simulink model "laneChangeOutputFeedback"  (R2019a)
settings: Solver=VariableStepAuto  StartTime=0.0  StopTime=60  RelTol=1e-3
values from neighbouring files (symbols this model uses):
  A = [-2 -timeHeadway 0]    [Controller.m]    (also in SimulinkScenario.m = [1 0 0;beta1 1 0; beta0 beta1 1; 0 beta0 beta1; 0 0 beta0])
  B = [0; b1; 0; b2]    [SimulinkScenario.m]
  C = [1 timeHeadway 0; 0 1 timeHeadway; 0 0 1]    [Controller.m]    (also in SimulinkScenario.m = [1 0 0 0])
  Cf = 12e3    (= 12000)    [sim_parameters.m]
  Cr = 11e3    (= 11000)    [sim_parameters.m]
  inputTau = 1    [SimulinkScenario.m]
  Iz = 4000    [sim_parameters.m]
  Kd = K(1)    [SimulinkScenario.m]
  Ki = K(3)    [SimulinkScenario.m]
  Kp = K(2)    [SimulinkScenario.m]
  lf = 1.4    [sim_parameters.m]
  lr = 1.6    [sim_parameters.m]
  maxDelta = 25*pi/180    (= 0.436332312999)    [sim_parameters.m]
  maxDeltaDot = 9.4*pi/180    (= 0.164060949687)    [sim_parameters.m]
  vehMass = 2000    [sim_parameters.m]
  vxRef = 20    [SimulinkScenario.m]
libraries: autolibshared x2, simulink x1
settings Model: Creator=Fernando VM  LastModifiedBy=Fernando VM

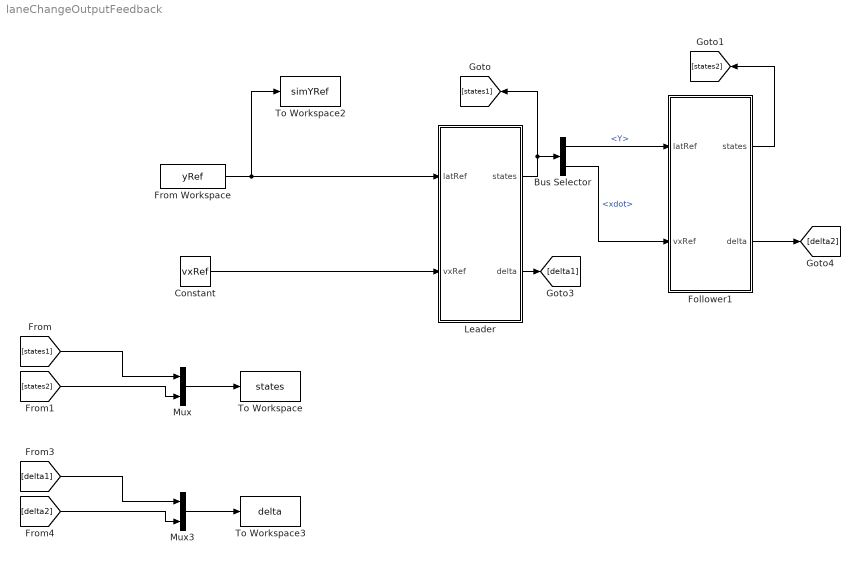
== system laneChangeOutputFeedback ==
  Bus Selector : BusSelector  OutputSignals=Y,xdot
  Constant : Constant  Value=vxRef
  Follower1 : Subsystem  mask{maxDelta=maxDelta, maxDeltaDot=maxDeltaDot, vehMass=vehMass, lf=lf, lr=lr, Cf=Cf, Cr=Cr, Iz=Iz, initPos=0, initVel=20, A=A, B=B, C=C, Kp=Kp, Ki=Ki, Kd=Kd, inputTau=inputTau}
      mask prompts: maxDelta "Max Delta"; maxDeltaDot "Max Delta Variation"; vehMass "Vehicle Mass"; lf "Dist Center of Mass to Front Axle"; lr "Dist Center of Mass to Rear Axle"; Cf "Front Tire Stiffness"; Cr "Rear Tire Sitffness"; Iz "Yaw Inertia"; initPos "Initial Long Position"; initVel "Initial Long Velocity"; inputTau "Input filter time constant"
      mask DialogControl ParameterGroupVar Prompt: Vehicle Parameters
      mask DialogControl Container6 Prompt: Initial Conditions
      mask DialogControl Container3 Prompt: Linear Model
      mask DialogControl Container5 Prompt: Controller
  From Workspace : FromWorkspace  VariableName=yRef  SampleTime=0
  Leader : Subsystem  mask{maxDelta=maxDelta, maxDeltaDot=maxDeltaDot, vehMass=vehMass, lf=lf, lr=lr, Cf=Cf, Cr=Cr, Iz=Iz, initPos=9.71, initVel=20, A=A, B=B, C=C, Kp=Kp, Ki=Ki, Kd=Kd, inputTau=inputTau}
      mask prompts: maxDelta "Max Delta"; maxDeltaDot "Max Delta Variation"; vehMass "Vehicle Mass"; lf "Dist Center of Mass to Front Axle"; lr "Dist Center of Mass to Rear Axle"; Cf "Front Tire Stiffness"; Cr "Rear Tire Sitffness"; Iz "Yaw Inertia"; initPos "Initial Long Position"; initVel "Initial Long Velocity"; inputTau "Input filter time constant"
      mask DialogControl ParameterGroupVar Prompt: Vehicle Parameters
      mask DialogControl Container6 Prompt: Initial Conditions
      mask DialogControl Container3 Prompt: Linear Model
      mask DialogControl Container5 Prompt: Controller
  Mux : Mux  Inputs=2
  Mux3 : Mux  Inputs=2
  To Workspace : ToWorkspace  VariableName=states  SampleTime=-1
  To Workspace2 : ToWorkspace  VariableName=simYRef  SampleTime=-1
  To Workspace3 : ToWorkspace  VariableName=delta  SampleTime=-1
  wires:
  From Workspace/1 -> Leader/1(latRef), To Workspace2/1
  Constant/1 -> Leader/2(vxRef)
  Leader/1(states) -> [states1], Bus Selector/1
  Bus Selector/2 -> Follower1/2(vxRef)  "<xdot>"
  Follower1/2(delta) -> [delta2]
  Follower1/1(states) -> [states2]
  Mux/1 -> To Workspace/1
  [states1] -> Mux/1
  [states2] -> Mux/2
  Leader/2(delta) -> [delta1]
  [delta2] -> Mux3/2
  [delta1] -> Mux3/1
  Mux3/1 -> To Workspace3/1
  Bus Selector/1 -> Follower1/1(latRef)  "<Y>"

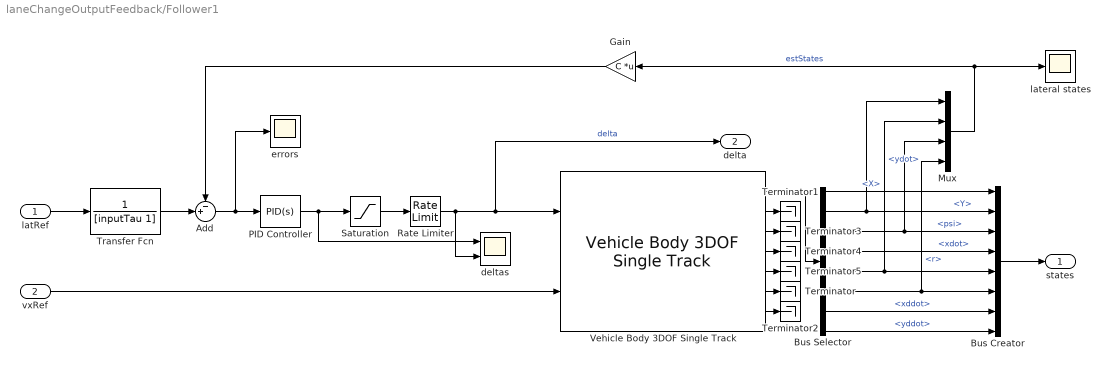
== system laneChangeOutputFeedback/Follower1 ==
  latRef : Inport
  vxRef : Inport  Port=2
  Add : Sum  Inputs=-+|
  Bus Creator : BusCreator  Inputs=8
  Bus Selector : BusSelector  OutputSignals=InertFrm.Cg.Disp.X,InertFrm.Cg.Disp.Y,InertFrm.Cg.Ang.psi,BdyFrm.Cg.Vel.xdot,BdyFrm.Cg.Vel.ydot,BdyFrm.Cg.AngVel.r,BdyFrm.Cg.Acc.xddot,BdyFrm.Cg.Acc.yddot
  Gain : Gain  Gain=C  Multiplication=Matrix(K*u)
  Mux : Mux
  PID Controller : simulink/Continuous/PID Controller  Controller=PID  Form=Parallel  TimeDomain=Continuous-time  SampleTime=-1  IntegratorMethod=Forward Euler  FilterMethod=Forward Euler  ControllerParametersSource=internal  P=Kp  I=Ki  D=Kd  UseFilter=on  N=100  TunerSelectOption=Transfer Function Based (PID Tuner App)  InitialConditionSource=internal  InitialConditionForIntegrator=0  InitialConditionForFilter=0  DifferentiatorICPrevScaledInput=0  ExternalReset=none  TrackingMode=off  Kt=1  LimitOutput=off  UpperSaturationLimit=inf  LowerSaturationLimit=-inf  LinearizeAsGain=on  AntiWindupMode=none  Kb=1  POutMin=[]  POutMax=[]  IOutMin=[]  IOutMax=[]  DOutMin=[]  DOutMax=[]  NOutMin=[]  NOutMax=[]  SumOutMin=[]  SumOutMax=[]  SaturationOutMin=[]  SaturationOutMax=[]  PParamMin=[]  PParamMax=[]  IParamMin=[]  IParamMax=[]  DParamMin=[]  DParamMax=[]  NParamMin=[]  NParamMax=[]  KbParamMin=[]  KbParamMax=[]  KtParamMin=[]  KtParamMax=[]  KbOutMin=[]  KbOutMax=[]  KtOutMin=[]  KtOutMax=[]  IntegratorOutMin=[]  IntegratorOutMax=[]  FilterOutMin=[]  FilterOutMax=[]  SumI1OutMin=[]  SumI1OutMax=[]  SumI2OutMin=[]  SumI2OutMax=[]  SumI3OutMin=[]  SumI3OutMax=[]  SumI4OutMin=[]  SumI4OutMax=[]  SumDOutMin=[]  SumDOutMax=[]  DifferentiatorOutMin=[]  DifferentiatorOutMax=[]  FilterDiffOutCoefMin=[]  FilterDiffOutCoefMax=[]  ReciprocalOutMin=[]  ReciprocalOutMax=[]  SumDenOutMin=[]  SumDenOutMax=[]  SumNumOutMin=[]  SumNumOutMax=[]  DivideOutMin=[]  DivideOutMax=[]  IntegratorContinuousStateAttributes=''  IntegratorStateMustResolveToSignalObject=off  IntegratorRTWStateStorageClass=Auto  FilterContinuousStateAttributes=''  FilterStateMustResolveToSignalObject=off  FilterRTWStateStorageClass=Auto  ParallelPVariant=InternalParameters  IdealPVariant=Disabled  IVariant=InternalParameters  DVariant=InternalParameters  IntegratorVariant=Continuous  SatVariant=Disabled  AWVariant=Passthrough  PCopyVariant=Disabled  TRVariant=Disabled  FdbkBlocksVariant=Forward  IdealPFdbkVariant=Disabled  SatFdbkVariant=Disabled  DerivativeFilterVariant=ContFilter  NVariant=InternalParameters  NCopyVariant=Disabled  FilterICVariant=InternalICsFilter  IntegratorICVariant=InternalICs  ExternalResetVariant=Disabled  TRSumVariant=Passthrough  SumFdbkVariant=Disabled  SumVariant=Sum_PID
  Rate Limiter : RateLimiter  RisingSlewLimit=maxDeltaDot  FallingSlewLimit=-maxDeltaDot  SampleTimeMode=inherited
  Saturation : Saturate  UpperLimit=maxDelta  LowerLimit=-maxDelta
  Terminator{,1..5} (6 alike) : Terminator
  Transfer Fcn : TransferFcn  Denominator=[inputTau 1]
  Vehicle Body 3DOF Single Track : autolibshared/Vehicle Body 3DOF Single Track  trackMode=Single (bicycle)  inputMode=External longitudinal velocity  frontSteerMode=on  rearSteerMode=off  windMode=off  muMode=off  extFMode=off  extMMode=off  extXo=off  extpsio=off  extxdoto=off  extro=off  extYo=off  extTamb=off  extydoto=off  aMode=2  NF=2  NR=2  m=vehMass  a=lf  b=lr  h=0.35  X_o=initPos  xdot_o=0  CalphaMode=off  sigmaMode=on  d=0  w=[1.4,1.4]  Cy_f=Cf  Cy_r=Cr  sigma_f=.1  sigma_r=.1  alpha_f_brk=[-.1 .1]  Cy_f_data=[-9e3 9e3]  alpha_r_brk=[-.1 .1]  Cy_r_data=[-9e3 9e3]  Y_o=0  ydot_o=0  Izz=Iz  psi_o=0  r_o=0  Af=2  Cd=.3  Cl=.1  Cpm=.1  beta_w=[0:0.01:0.3]  Cs=[0:0.03:0.9]  Cym=[0:0.01:0.3]  Pabs=101325  Tair=273  g=9.81  mu=1  xdot_tol=.01  Fznom=5000  Fxtire_sat=7e4  Fytire_sat=7e4  longOff=0  latOff=0  vertOff=0  wrapAng=off
      settings: SourceProductName=Powertrain Blockset  SourceProductBaseCode=PW
  deltas : Scope  NumInputPorts=2
  errors : Scope
  lateral states : Scope
  states : Outport
  delta : Outport  Port=2
  wires:
  Add/1 -> PID Controller/1, errors/1
  PID Controller/1 -> deltas/1, Saturation/1
  Vehicle Body 3DOF Single Track/1 -> Bus Selector/1
  Bus Selector/2 -> Bus Creator/2, Mux/1  "<Y>"
  Rate Limiter/1 -> delta/1, Vehicle Body 3DOF Single Track/1, deltas/2  "delta"
  Saturation/1 -> Rate Limiter/1
  vxRef/1 -> Vehicle Body 3DOF Single Track/2
  Mux/1 -> Gain/1, lateral states/1  "estStates"
  latRef/1 -> Transfer Fcn/1
  Transfer Fcn/1 -> Add/2
  Vehicle Body 3DOF Single Track/2 -> Terminator1/1
  Vehicle Body 3DOF Single Track/6 -> Terminator/1
  Vehicle Body 3DOF Single Track/7 -> Terminator2/1
  Bus Selector/5 -> Bus Creator/5, Mux/2  "<ydot>"
  Bus Selector/3 -> Bus Creator/3, Mux/3  "<psi>"
  Bus Selector/6 -> Bus Creator/6, Mux/4  "<r>"
  Vehicle Body 3DOF Single Track/3 -> Terminator3/1
  Vehicle Body 3DOF Single Track/4 -> Terminator4/1
  Vehicle Body 3DOF Single Track/5 -> Terminator5/1
  Bus Creator/1 -> states/1
  Bus Selector/1 -> Bus Creator/1  "<X>"
  Bus Selector/4 -> Bus Creator/4  "<xdot>"
  Bus Selector/7 -> Bus Creator/7  "<xddot>"
  Bus Selector/8 -> Bus Creator/8  "<yddot>"
  Gain/1 -> Add/1

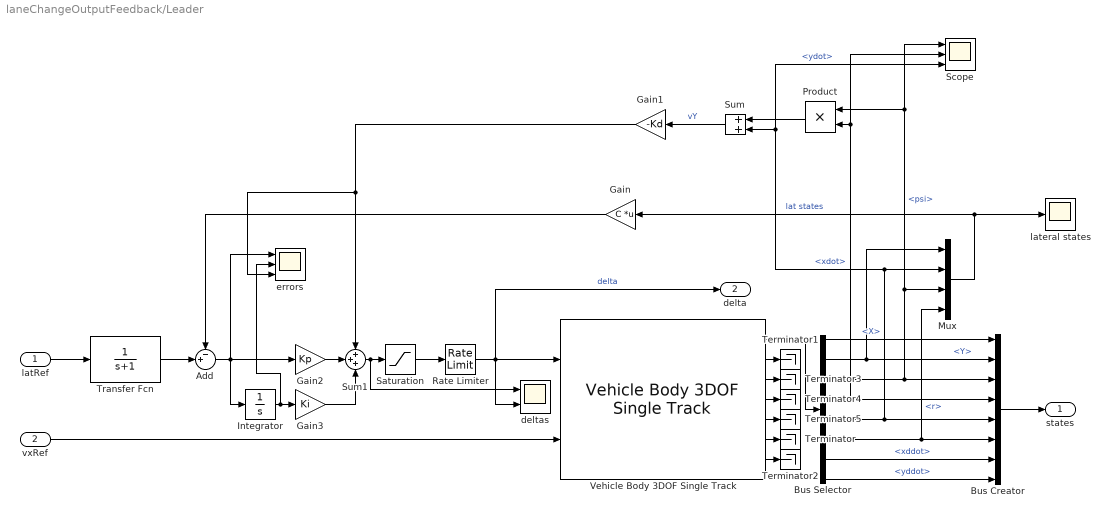
== system laneChangeOutputFeedback/Leader ==
  latRef : Inport
  vxRef : Inport  Port=2
  Add : Sum  Inputs=-+|
  Bus Creator : BusCreator  Inputs=8
  Bus Selector : BusSelector  OutputSignals=InertFrm.Cg.Disp.X,InertFrm.Cg.Disp.Y,InertFrm.Cg.Ang.psi,BdyFrm.Cg.Vel.xdot,BdyFrm.Cg.Vel.ydot,BdyFrm.Cg.AngVel.r,BdyFrm.Cg.Acc.xddot,BdyFrm.Cg.Acc.yddot
  Gain : Gain  Gain=C  Multiplication=Matrix(K*u)
  Gain1 : Gain  Gain=-Kd
  Gain2 : Gain  Gain=Kp
  Gain3 : Gain  Gain=Ki
  Integrator : Integrator
  Mux : Mux
  Product : Product
  Rate Limiter : RateLimiter  RisingSlewLimit=maxDeltaDot  FallingSlewLimit=-maxDeltaDot  SampleTimeMode=inherited
  Saturation : Saturate  UpperLimit=maxDelta  LowerLimit=-maxDelta
  Scope : Scope  NumInputPorts=3
  Sum : Sum
  Sum1 : Sum  Inputs=+++
  Terminator{,1..5} (6 alike) : Terminator
  Transfer Fcn : TransferFcn  Denominator=[1 1]
  Vehicle Body 3DOF Single Track : autolibshared/Vehicle Body 3DOF Single Track  trackMode=Single (bicycle)  inputMode=External longitudinal velocity  frontSteerMode=on  rearSteerMode=off  windMode=off  muMode=off  extFMode=off  extMMode=off  extXo=off  extpsio=off  extxdoto=off  extro=off  extYo=off  extTamb=off  extydoto=off  aMode=2  NF=2  NR=2  m=vehMass  a=lf  b=lr  h=0.35  X_o=initPos  xdot_o=0  CalphaMode=off  sigmaMode=on  d=0  w=[1.4,1.4]  Cy_f=Cf  Cy_r=Cr  sigma_f=.1  sigma_r=.1  alpha_f_brk=[-.1 .1]  Cy_f_data=[-9e3 9e3]  alpha_r_brk=[-.1 .1]  Cy_r_data=[-9e3 9e3]  Y_o=0  ydot_o=0  Izz=Iz  psi_o=0  r_o=0  Af=2  Cd=.3  Cl=.1  Cpm=.1  beta_w=[0:0.01:0.3]  Cs=[0:0.03:0.9]  Cym=[0:0.01:0.3]  Pabs=101325  Tair=273  g=9.81  mu=1  xdot_tol=.01  Fznom=5000  Fxtire_sat=7e4  Fytire_sat=7e4  longOff=0  latOff=0  vertOff=0  wrapAng=off
      settings: SourceProductName=Powertrain Blockset  SourceProductBaseCode=PW
  deltas : Scope  NumInputPorts=2
  errors : Scope  NumInputPorts=3
  lateral states : Scope
  states : Outport
  delta : Outport  Port=2
  wires:
  Add/1 -> Integrator/1, Gain2/1, errors/1
  Vehicle Body 3DOF Single Track/1 -> Bus Selector/1
  Bus Selector/2 -> Bus Creator/2, Mux/1  "<Y>"
  Rate Limiter/1 -> deltas/2, delta/1, Vehicle Body 3DOF Single Track/1  "delta"
  Saturation/1 -> Rate Limiter/1
  vxRef/1 -> Vehicle Body 3DOF Single Track/2
  Mux/1 -> Gain/1, lateral states/1  "lat states"
  latRef/1 -> Transfer Fcn/1
  Transfer Fcn/1 -> Add/2
  Vehicle Body 3DOF Single Track/2 -> Terminator1/1
  Vehicle Body 3DOF Single Track/6 -> Terminator/1
  Vehicle Body 3DOF Single Track/7 -> Terminator2/1
  Bus Selector/5 -> Bus Creator/5, Scope/3, Sum/2, Mux/2  "<ydot>"
  Bus Selector/3 -> Bus Creator/3, Scope/1, Product/1, Mux/3  "<psi>"
  Bus Selector/6 -> Bus Creator/6, Mux/4  "<r>"
  Vehicle Body 3DOF Single Track/3 -> Terminator3/1
  Vehicle Body 3DOF Single Track/4 -> Terminator4/1
  Vehicle Body 3DOF Single Track/5 -> Terminator5/1
  Bus Creator/1 -> states/1
  Bus Selector/1 -> Bus Creator/1  "<X>"
  Bus Selector/4 -> Scope/2, Product/2, Bus Creator/4  "<xdot>"
  Bus Selector/7 -> Bus Creator/7  "<xddot>"
  Bus Selector/8 -> Bus Creator/8  "<yddot>"
  Gain/1 -> Add/1
  Product/1 -> Sum/1
  Sum/1 -> Gain1/1  "vY"
  Integrator/1 -> errors/2, Gain3/1
  Gain2/1 -> Sum1/2
  Sum1/1 -> deltas/1, Saturation/1
  Gain3/1 -> Sum1/3
  Gain1/1 -> errors/3, Sum1/1
